simulink model "dynamic_APF"  (R2022b)
settings: Solver=VariableStepAuto  StartTime=0.0  StopTime=inf  RelTol=1e-3
InitFcn:
  | %% INITIALIZATION
  | 
  | %% UAV PARAMETERS
  | 
  | mass = 1.2;
  | Ib = diag([1.2416 1.2416 2*1.2416]);
  | 
  | %% SAMPLING TIME
  | Ts=0.001;
  | 
  | %% PLANNER
  | t_iniz = 0;
  | ttot=20; %duration
  | tdead=10; %dead time to evaluate the steady-state
  | tot_time = ttot + tdead;
  | t1=linspace(0,ttot,round(ttot/Ts));
  | t=linspace(0,ttot+tdead,round(ttot/Ts)+round(tdead/Ts));
  | p= zeros(4,length(t1)); dot_p= zeros(4,length(t1)); ddot_p= zeros(4,length(t1));
  | p_d= zeros(4,length(t)); dot_p_d= zeros(4,length(t)); ddot_p_d= zeros(4,length(t));
  | %Initial and final conditions
  | x0= 0; xf=1; dot_x0= 0; dot_xf=0; ddot_x0=0; ddot_xf=0; dddot_x0 = 0; dddot_xf = 0;
  | y0= 0; yf=1; dot_y0= 0; dot_yf=0; ddot_y0=0; ddot_yf=0; dddot_y0 = 0; dddot_yf = 0;
  | z0= -1; zf=-4; dot_z0= 0; dot_zf=0; ddot_z0=0; ddot_zf=0; dddot_z0 = 0; dddot_zf = 0;
  | psi0 = 0;
  | psif=deg2rad(20); dot_psi0= 0; dot_psif=0; ddot_psi0=0; ddot_psif=0; dddot_psi0 = 0; dddot_psif = 0;
  | p0=[x0,y0,z0,psi0]; dot_p0=[dot_x0,dot_y0,dot_z0,dot_psi0]; ddot_p0=[ddot_x0,ddot_y0,ddot_z0,ddot_psi0]; dddot_p0=[dddot_x0,dddot_y0,dddot_z0,dddot_psi0];
  | pf=[xf,yf,zf,psif]; dot_pf=[dot_xf,dot_yf,dot_zf,dot_psif]; ddot_pf=[ddot_xf,ddot_yf,ddot_zf,ddot_psif]; dddot_pf=[dddot_xf,dddot_yf,dddot_zf,dddot_psif];
  | %5-th order polynomial
  | a0=zeros(1,4); a1=zeros(1,4); a2=zeros(1,4); a3=zeros(1,4); a4=zeros(1,4); a5=zeros(1,4); a6 = zeros(1,4); a7 = zeros(1,4);
  | 
  | for j=1:4
  |     A = [t_iniz^7, t_iniz^6, t_iniz^5, t_iniz^4, t_iniz^3, t_iniz^2, t_iniz, 1;
  |         ttot^7, ttot^6, ttot^5, ttot^4, ttot^3, ttot^2, ttot, 1;
  |         7*t_iniz^6, 6*t_iniz^5, 5*t_iniz^4, 4*t_iniz^3, 3*t_iniz^2, 2*t_iniz, 1, 0;
  |         7*ttot^6, 6*ttot^5, 5*ttot^4, 4*ttot^3, 3*ttot^2, 2*ttot, 1, 0;
  |         42*t_iniz^5, 30*t_iniz^4, 20*t_iniz^3, 12*t_iniz^2, 6*t_iniz, 2, 0, 0;
  |         42*ttot^5, 30*ttot^4, 20*ttot^3, 12*ttot^2, 6*ttot, 2, 0, 0;
  |         210*t_iniz^4, 120*t_iniz^3, 60*t_iniz^2, 24*t_iniz, 6, 0, 0, 0;
  |         210*ttot^4, 120*ttot^3, 60*ttot^2, 24*ttot, 6, 0, 0, 0];
  |     b = [p0(j) pf(j) dot_p0(j) dot_pf(j) ddot_p0(j) ddot_pf(j) dddot_p0(j) dddot_pf(j)]';
  |     a_temp = A\b;
  |     a7(j) = a_temp(1);
  |     a6(j) = a_temp(2);
  |     a5(j) = a_temp(3);
  |     a4(j) = a_temp(4);
  |     a3(j) = a_temp(5);
  |     a2(j) = a_temp(6);
  |     a1(j) = a_temp(7);
  |     a0(j) = a_temp(8);
  | 
  |     %trajectories
  |     p(j,:)=a7(j)*t1.^7 + a6(j)*t1.^6 + a5(j)*t1.^5 +a4(j)*t1.^4 +a3(j)*t1.^3 +a2(j)*t1.^2 +a1(j)*t1 +a0(j);
  |     dot_p(j,:) = 7*a7(j)*t1.^6 + 6*a6(j)*t1.^5 + 5*a5(j)*t1.^4 +4*a4(j)*t1.^3 +3*a3(j)*t1.^2 +2*a2(j)*t1 +a1(j);
  |     ddot_p(j,:) = 42*a7(j)*t1.^5 + 30*a6(j)*t1.^4 + 5*4*a5(j)*t1.^3 +4*3*a4(j)*t1.^2 +3*2*a3(j)*t1 +2*a2(j);
  |     %addition of the stead-state terms
  |     p_d(j,:)=[p(j,:) zeros(1,round(tdead/Ts))+pf(j)];
  |     dot_p_d(j,:)=[dot_p(j,:) zeros(1,round(tdead/Ts))+dot_pf(j)];
  |     ddot_p_d(j,:)=[ddot_p(j,:) zeros(1,round(tdead/Ts))+ddot_pf(j)];
  | end
  | %data for Simulink
  | %pos_0 = [x0 y0 z0];
  | pos_0 = [0 0 0];
  | lin_vel_0 = [dot_x0 dot_y0 dot_z0];
  | w_bb_0 = [0 0 0];
  | csi_d=p_d(1:3,:); dot_csi_d=dot_p_d(1:3,:); ddot_csi_d=ddot_p_d(1:3,:);
  | psi_d=p_d(4,:); dot_psi_d=dot_p_d(4,:); ddot_psi_d=ddot_p_d(4,:);
undefined symbols (not defined in the file): k_att, k_rep, kp, kr, kv, kw
libraries: robotcorelib x1, simulink x1, uavutilslib x1
settings Model: Creator=fabioruggiero  LastModifiedBy=stefa
settings OptimizationCC: ReuseModelBlockBuffer=on
settings ModelReferenceCC: EnableRefExpFcnMdlSchedulingChecks=on

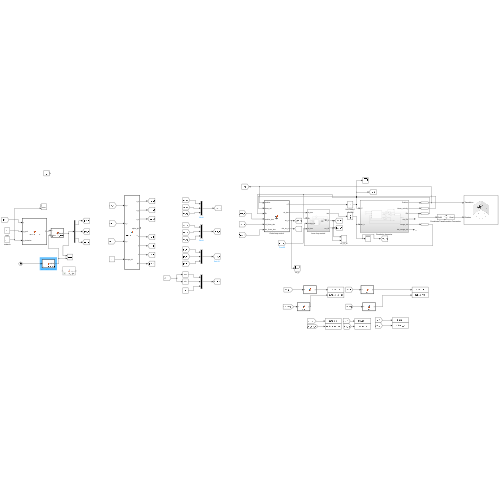
[thumbnail: Simulink's stored preview of the top-level diagram]
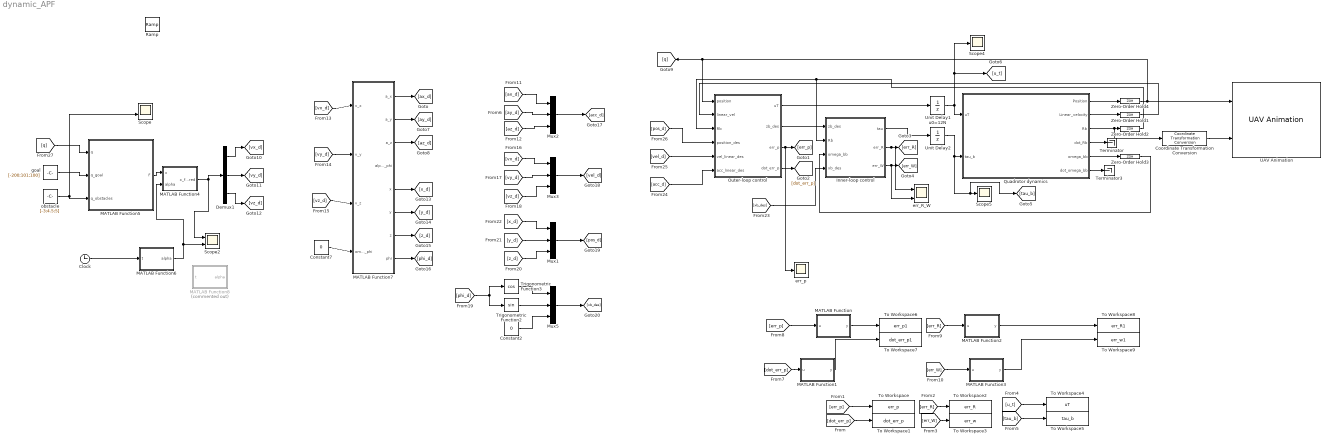
== system dynamic_APF ==
  Clock : Clock
  Constant2 : Constant  Value=0
  Constant7 : Constant  Value=0
  Coordinate Transformation Conversion : robotcorelib/Coordinate Transformation Conversion  InputRepresentation=Rotation Matrix  InputEulerSequence=ZYX  ShowTrVecInputPort=on  OutputRepresentation=Quaternion  OutputEulerSequence=ZYX  ShowTrVecOutputPort=on  SimulateUsing=Interpreted execution
  Demux1 : Demux  Outputs=3
  Inner-loop control : Subsystem
  MATLAB Function : MATLAB Function  TreatAsAtomicUnit=on
  MATLAB Function1 : MATLAB Function  TreatAsAtomicUnit=on
  MATLAB Function2 : MATLAB Function  TreatAsAtomicUnit=on
  MATLAB Function3 : MATLAB Function  TreatAsAtomicUnit=on
  MATLAB Function4 : MATLAB Function  TreatAsAtomicUnit=on
  MATLAB Function5 : MATLAB Function  TreatAsAtomicUnit=on
  MATLAB Function6 : MATLAB Function  TreatAsAtomicUnit=on
  MATLAB Function7 : MATLAB Function  TreatAsAtomicUnit=on
  MATLAB Function8 : MATLAB Function  Commented=on  TreatAsAtomicUnit=on
  Mux{1..3,5} (4 alike) : Mux  Inputs=3
  Outer-loop control : MATLAB Function  TreatAsAtomicUnit=on
  Quadrotor dynamics : Subsystem
  Ramp : simulink/Sources/Ramp  slope=1  start=0  InitialOutput=0
  Scope : Scope  NumInputPorts=2
  Scope2 : Scope  NumInputPorts=2
  Scope4 : Scope
  Scope5 : Scope
  Terminator : Terminator
  Terminator3 : Terminator
  To Workspace : ToWorkspace  VariableName=err_p  SaveFormat=Timeseries  SampleTime=-1
  To Workspace1 : ToWorkspace  VariableName=dot_err_p  SaveFormat=Timeseries  SampleTime=-1
  To Workspace2 : ToWorkspace  VariableName=err_R  SaveFormat=Timeseries  SampleTime=-1
  To Workspace3 : ToWorkspace  VariableName=err_w  SaveFormat=Timeseries  SampleTime=-1
  To Workspace4 : ToWorkspace  VariableName=uT  SaveFormat=Timeseries  SampleTime=-1
  To Workspace5 : ToWorkspace  VariableName=tau_b  SaveFormat=Timeseries  SampleTime=-1
  To Workspace6 : ToWorkspace  VariableName=err_p1  SaveFormat=Timeseries  SampleTime=-1
  To Workspace7 : ToWorkspace  VariableName=dot_err_p1  SaveFormat=Timeseries  SampleTime=-1
  To Workspace8 : ToWorkspace  VariableName=err_R1  SaveFormat=Timeseries  SampleTime=-1
  To Workspace9 : ToWorkspace  VariableName=err_w1  SaveFormat=Timeseries  SampleTime=-1
  Trigonometric Function2 : Trigonometry
  Trigonometric Function3 : Trigonometry  Operator=cos
  UAV Animation : uavutilslib/UAV Animation  UAVType=Multirotor  UAVSize=1  InertialZDirection=Down  SampleTime=0.01
  Unit Delay1 u0=12N : UnitDelay  InitialCondition=11.77  SampleTime=Ts
  Unit Delay2 : UnitDelay  InitialCondition=[0 0 0]  SampleTime=Ts
  Zero-Order Hold{1..4} (4 alike) : ZeroOrderHold  SampleTime=Ts
  err_R_W : Scope  NumInputPorts=2
  err_p : Scope
  goal : Constant  Value=[-200;101;100]
  obstacle : Constant  Value=[-3;4.5;5]
  wires:
  Outer-loop control/1(uT) -> Unit Delay1 u0=12N/1
  Unit Delay1 u0=12N/1 -> Quadrotor dynamics/1(uT), Scope4/1, [u_t]
  Quadrotor dynamics/1(Position) -> Zero-Order Hold4/1
  Quadrotor dynamics/2(Linear_velocity) -> Zero-Order Hold1/1
  Quadrotor dynamics/3(Rb) -> Coordinate Transformation Conversion/1, Zero-Order Hold2/1
  Quadrotor dynamics/5(omega_bb) -> Zero-Order Hold3/1
  Zero-Order Hold1/1 -> Outer-loop control/2(linear_vel)
  Zero-Order Hold2/1 -> Outer-loop control/3(Rb), Inner-loop control/2(Rb)
  Quadrotor dynamics/4(dot_Rb) -> Terminator/1
  Outer-loop control/3(err_p) -> err_p/1, [err_p]
  Outer-loop control/4(dot_err_p) -> [dot_err_p]
  Quadrotor dynamics/6(dot_omega_bb) -> Terminator3/1
  Coordinate Transformation Conversion/1 -> UAV Animation/2
  Outer-loop control/2(zb_des) -> Inner-loop control/1(zb_des)
  Zero-Order Hold3/1 -> Inner-loop control/3(omega_bb)
  Inner-loop control/1(tau) -> Unit Delay2/1
  [dot_err_p] -> To Workspace1/1
  [err_p] -> To Workspace/1
  Inner-loop control/2(err_R) -> err_R_W/1, [err_R]
  Inner-loop control/3(err_W) -> err_R_W/2, [err_W]
  [err_R] -> To Workspace2/1
  [err_W] -> To Workspace3/1
  Unit Delay2/1 -> [tau_b], Scope5/1, Quadrotor dynamics/2(tau_b)
  [u_t] -> To Workspace4/1
  [tau_b] -> To Workspace5/1
  [err_R] -> MATLAB Function2/1(u)
  [dot_err_p] -> MATLAB Function1/1(u)
  [err_p] -> MATLAB Function/1(u)
  [err_W] -> MATLAB Function3/1(u)
  MATLAB Function/1(y) -> To Workspace6/1
  MATLAB Function1/1(y) -> To Workspace7/1
  MATLAB Function2/1(y) -> To Workspace8/1
  MATLAB Function3/1(y) -> To Workspace9/1
  obstacle/1 -> Scope/2, MATLAB Function5/3(q_obstacles)
  Zero-Order Hold4/1 -> UAV Animation/1, [q], Outer-loop control/1(position)
  goal/1 -> MATLAB Function5/2(q_goal)
  Constant2/1 -> Mux5/3
  Trigonometric Function3/1 -> Mux5/1
  Trigonometric Function2/1 -> Mux5/2
  Constant7/1 -> MATLAB Function7/4(omega_phi)
  MATLAB Function7/1(a_x) -> [ax_d]
  MATLAB Function7/2(a_y) -> [ay_d]
  MATLAB Function7/3(a_z) -> [az_d]
  [ay_d] -> Mux2/2
  [ax_d] -> Mux2/1
  [az_d] -> Mux2/3
  Demux1/1 -> [vx_d]
  Demux1/2 -> [vy_d]
  Demux1/3 -> [vz_d]
  [vx_d] -> MATLAB Function7/1(v_x)
  [vy_d] -> MATLAB Function7/2(v_y)
  [vz_d] -> MATLAB Function7/3(v_z)
  [vx_d] -> Mux3/1
  [vy_d] -> Mux3/2
  [vz_d] -> Mux3/3
  MATLAB Function7/5(x) -> [x_d]
  MATLAB Function7/6(y) -> [y_d]
  MATLAB Function7/7(z) -> [z_d]
  MATLAB Function7/8(phi) -> [phi_d]
  [phi_d] -> Trigonometric Function2/1, Trigonometric Function3/1
  [z_d] -> Mux1/3
  [y_d] -> Mux1/2
  [x_d] -> Mux1/1
  Mux2/1 -> [acc_d]
  Mux3/1 -> [vel_d]
  Mux1/1 -> [pos_d]
  Mux5/1 -> [xb_des]
  [xb_des] -> Inner-loop control/4(xb_des)
  [acc_d] -> Outer-loop control/6(acc_linear_des)
  [vel_d] -> Outer-loop control/5(vel_linear_des)
  [pos_d] -> Outer-loop control/4(position_des)
  [q] -> MATLAB Function5/1(q)
  MATLAB Function5/1(F) -> MATLAB Function4/1(x)
  MATLAB Function4/1(x_filtered) -> Demux1/1, Scope2/1
  Clock/1 -> MATLAB Function6/1(t)
  MATLAB Function6/1(alpha) -> Scope2/2, MATLAB Function4/2(alpha)

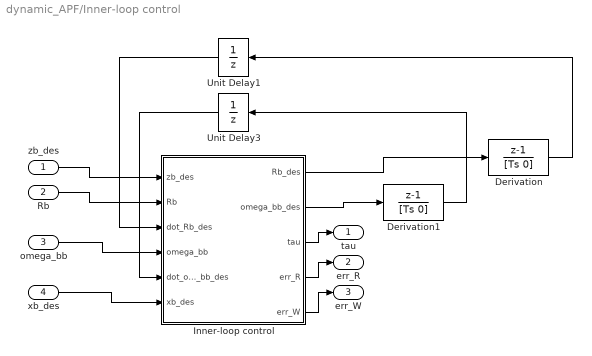
== system dynamic_APF/Inner-loop control ==
  zb_des : Inport
  Rb : Inport  Port=2
  omega_bb : Inport  Port=3
  xb_des : Inport  Port=4
  Derivation : DiscreteTransferFcn  Numerator=[1 -1]  Denominator=[Ts 0]  InitialStates=[1 0 0;0 1 0;0 0 1]  SampleTime=Ts
  Derivation1 : DiscreteTransferFcn  Numerator=[1 -1]  Denominator=[Ts 0]  InitialStates=[0 0 0]  SampleTime=Ts
  Inner-loop control : MATLAB Function  TreatAsAtomicUnit=on
  Unit Delay1 : UnitDelay  InitialCondition=eye(3)  SampleTime=Ts
  Unit Delay3 : UnitDelay  InitialCondition=[0 0 0]  SampleTime=Ts
  tau : Outport
  err_R : Outport  Port=2
  err_W : Outport  Port=3
  wires:
  xb_des/1 -> Inner-loop control/6(xb_des)
  Inner-loop control/4(err_R) -> err_R/1
  Rb/1 -> Inner-loop control/2(Rb)
  Inner-loop control/3(tau) -> tau/1
  Unit Delay1/1 -> Inner-loop control/3(dot_Rb_des)
  Derivation1/1 -> Unit Delay3/1
  Inner-loop control/5(err_W) -> err_W/1
  Unit Delay3/1 -> Inner-loop control/5(dot_omega_bb_des)
  Derivation/1 -> Unit Delay1/1
  zb_des/1 -> Inner-loop control/1(zb_des)
  omega_bb/1 -> Inner-loop control/4(omega_bb)
  Inner-loop control/1(Rb_des) -> Derivation/1
  Inner-loop control/2(omega_bb_des) -> Derivation1/1

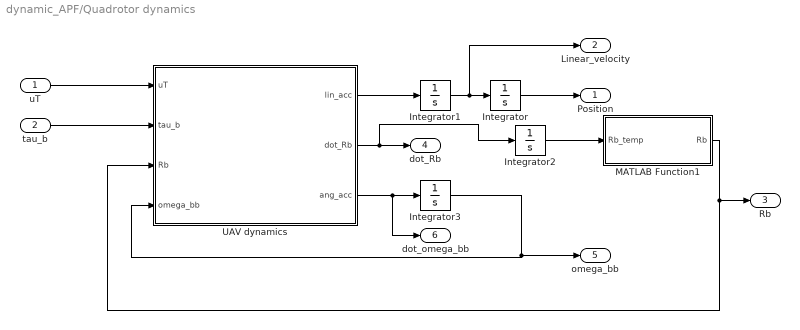
== system dynamic_APF/Quadrotor dynamics ==
  uT : Inport
  tau_b : Inport  Port=2
  Integrator : Integrator  InitialCondition=pos_0
  Integrator1 : Integrator  InitialCondition=lin_vel_0
  Integrator2 : Integrator  InitialCondition=[1 0 0; 0 1 0;0 0 1]
  Integrator3 : Integrator  InitialCondition=w_bb_0
  MATLAB Function1 : MATLAB Function  TreatAsAtomicUnit=on
  UAV dynamics : MATLAB Function  TreatAsAtomicUnit=on
  Position : Outport
  Linear_velocity : Outport  Port=2
  Rb : Outport  Port=3
  dot_Rb : Outport  Port=4
  omega_bb : Outport  Port=5
  dot_omega_bb : Outport  Port=6
  wires:
  tau_b/1 -> UAV dynamics/2(tau_b)
  Integrator/1 -> Position/1
  UAV dynamics/3(ang_acc) -> dot_omega_bb/1, Integrator3/1
  UAV dynamics/1(lin_acc) -> Integrator1/1
  uT/1 -> UAV dynamics/1(uT)
  Integrator1/1 -> Linear_velocity/1, Integrator/1
  Integrator3/1 -> UAV dynamics/4(omega_bb), omega_bb/1
  UAV dynamics/2(dot_Rb) -> Integrator2/1, dot_Rb/1
  MATLAB Function1/1(Rb) -> Rb/1, UAV dynamics/3(Rb)
  Integrator2/1 -> MATLAB Function1/1(Rb_temp)

== matlab function dynamic_APF/MATLAB Function2 ==
  data: u input; y output
function y = fcn(u)

y = norm(u);

== matlab function dynamic_APF/MATLAB Function3 ==
  data: u input; y output
function y = fcn(u)

y = norm(u);

== matlab function dynamic_APF/MATLAB Function4 ==
  settings: updateMethod=DISCRETE
  data: x input; x_filtered output; alpha input
function x_filtered = exponential_moving_average_vector(x, alpha)
    % Funzione per calcolare la media mobile esponenziale di un vettore colonna 3x1.
    % x: vettore colonna di ingresso 3x1
    % alpha: fattore di smorzamento (0 < alpha < 1)
    % x_filtered: vettore colonna filtrato 3x1
%E' lo stesso filtro che abbiamo fatto con Manfredi, la differenza è che
%alpha è tempo variante, varia in funzione esponenziale con il tempo. Se
%allontano l ostacolo nn ho problemi, tanto la Fmax dipende dai
%coefficienti, ma se vario i coefficienti posso dover ritararre il filtro(E' stato inserito per diminuire la trust iniziale)
    % Verifica che l'input x sia un vettore colonna 3x1
    if ~isequal(size(x), [3, 1])
        error('L''input x deve essere un vettore colonna 3x1.');
    end
    
    % Inizializza la variabile persistente
    persistent x_filtered_prev
    
    % Se è la prima chiamata, inizializza la variabile persistente
    if isempty(x_filtered_prev)
        x_filtered_prev = [0;0;0];
    end
    
    % Applica il filtro a media mobile esponenziale elemento per elemento
    x_filtered = (1 - alpha) * x_filtered_prev + alpha * x;
    
    % Aggiorna la variabile persistente
    x_filtered_prev = x_filtered;
end

== matlab function dynamic_APF/MATLAB Function5 ==
  data: q input; F output; q_goal input; q_obstacles input; k_att parameter; k_rep parameter
function F  = calculate_force(q, q_goal, q_obstacles, k_att, k_rep)
% Funzione per calcolare la forza totale F(q) utilizzando il metodo dei potenziali artificiali
% 
% Inputs:
%   q - Posizione attuale del UAV (3x1 vettore)
%   q_goal - Posizione del goal (3x1 vettore)
%   q_obstacles - Posizioni degli ostacoli (3xn matrice, dove n è il numero di ostacoli)
%   k_att - Coefficiente di attrazione (scalare)
%   k_rep - Coefficiente di repulsione (scalare)
%   d0 - Distanza di influenza degli ostacoli (scalare)
% 
% Output:
%   F - Forza totale (3x1 vettore)
q=-q;
k_a=k_att;

d0=2.5;
e_pos = q_goal - q;
%Ua_q= 1/2*k_att*norm(e_pos)
if(norm(e_pos)<1)
    f_a = k_a * e_pos;
else
    f_a = k_a * e_pos/norm(e_pos);
end
gamma=3;
 % Inizializza la forza repulsiva
F_rep = zeros(3, 1);

% Calcola la forza repulsiva per ciascun ostacolo
for i = 1:size(q_obstacles, 2)
    q_obs = q_obstacles(:, i);
    dist = norm(q - q_obs);
    
    if dist <= d0
        eta_q = dist;
        eta_q0 = d0;
        grad_eta_q = (q - q_obs) / dist;
        
        F_rep = F_rep + (k_rep/(eta_q^2))*(1/eta_q - 1/eta_q0)^(gamma-1) * grad_eta_q;
    end
end
F = -f_a - F_rep;
end

== matlab function dynamic_APF/MATLAB Function6 ==
  data: t input; alpha output
function alpha = calculate_alpha(t)
    % Calcola il valore di alpha in base all'istante temporale t
    
    % Define initial and final alpha values
    alpha_initial = 0.0000005;
    alpha_final = 0.5;
    
    % Define the time duration over which alpha should reach final value
    time_to_increase = 10;  % Increase alpha over 10 seconds
    alpha = alpha_initial * (100*t / 2)^2;
    % Calculate alpha based on a combination of slow start and faster growth
%     if t <= 2  % Slow start for the first 2 seconds
%         alpha = alpha_initial * (t / 2)^2;  % Quadratic ramp up
%     else
%         alpha = alpha_initial + (alpha_final - alpha_initial) * ((t - 2) / (time_to_increase - 2));
%     end
    
    % Ensure alpha is within bounds
    alpha = max(min(alpha, alpha_final), alpha_initial);
end

== matlab function dynamic_APF/MATLAB Function7 ==
  settings: updateMethod=DISCRETE
  data: a_x output; a_y output; a_z output; alpha_phi output; x output; v_x input; y output; v_y input; v_z input; omega_phi input; z output; phi output; Ts parameter double
function [a_x, a_y, a_z, alpha_phi, x, y, z, phi] = calculate_state(v_x, v_y, v_z, omega_phi, Ts)
    % Calcola le posizioni e le accelerazioni a partire dalle velocità
    % Inizializza le variabili persistenti
    persistent x_prev y_prev z_prev phi_prev
    persistent v_x_prev v_y_prev v_z_prev omega_phi_prev
    dt=Ts;
    % Se è la prima chiamata, inizializza le variabili persistenti
    if isempty(x_prev)
        x_prev = 0;
        y_prev = 0;
        z_prev = 0;
        phi_prev = 0;
        v_x_prev = 0;
        v_y_prev = 0;
        v_z_prev = 0;
        omega_phi_prev = 0;
    end
    
    % Calcola le posizioni integrando le velocità
    x = x_prev + v_x * dt;
    y = y_prev + v_y * dt;
    z = z_prev + v_z * dt;
    phi = phi_prev + omega_phi * dt;
    
    % Calcola le accelerazioni derivando le velocità
    a_x = (v_x - v_x_prev) / dt;
    a_y = (v_y - v_y_prev) / dt;
    a_z = (v_z - v_z_prev) / dt;
    alpha_phi = (omega_phi - omega_phi_prev) / dt;
    
    % Aggiorna le variabili persistenti
    x_prev = x;
    y_prev = y;
    z_prev = z;
    phi_prev = phi;
    v_x_prev = v_x;
    v_y_prev = v_y;
    v_z_prev = v_z;
    omega_phi_prev = omega_phi;
end

== matlab function dynamic_APF/MATLAB Function8 ==
  data: t input; alpha output
function alpha = calculate_alpha(t)
    % Calcola il valore di alpha in base all'istante temporale t
    
    % Define initial and final alpha values
    alpha_initial = 0.05;
    alpha_final = 1;
    
    % Define the time duration over which alpha should increase
    time_to_increase = 5;  % Increase alpha over 10 seconds
    
    % Calculate alpha based on linear interpolation
    if t <= time_to_increase
        alpha = alpha_initial + (alpha_final - alpha_initial) * (t / time_to_increase);
    else
        alpha = alpha_final;
    end
end

== matlab function dynamic_APF/MATLAB Function ==
  data: u input; y output
function y = fcn(u)

y = norm(u);

== matlab function dynamic_APF/Quadrotor dynamics/UAV dynamics ==
  data: uT input size=1; tau_b input size=3; lin_acc output size=3; Rb input size=[3,3]; omega_bb input size=3; dot_Rb output size=[3,3]; ang_acc output size=3; mass parameter size=1; Ib parameter size=[3,3]
function [lin_acc, dot_Rb, ang_acc] = fcn(uT,tau_b,Rb,omega_bb,mass, Ib)

lin_acc = 9.81*[0 0 1]'-(uT/mass)*Rb*[0 0 1]';
dot_Rb = Rb*skew(omega_bb);
ang_acc = inv(Ib)*(-skew(omega_bb)*Ib*omega_bb + tau_b);

end

function S = skew(v)
if(numel(v)~= 1)
S= [0 -v(3) v(2); 
    v(3) 0 -v(1);
    -v(2) v(1) 0];
else
S= zeros(3);
end
end

== matlab function dynamic_APF/Outer-loop control ==
  data: position input size=3; uT output size=1; linear_vel input size=3; Rb input size=[3,3]; zb_des output size=3; mass parameter size=1; position_des input size=3; vel_linear_des input size=3; acc_linear_des input size=3; err_p output size=3; dot_err_p output size=3; kp parameter; kv parameter
function [uT, zb_des, err_p, dot_err_p] = fcn(position, linear_vel, Rb, mass, ...
    position_des, vel_linear_des, acc_linear_des, kp, kv)

%% WRITE HERE THE OUTER-LOOP CONTROL
% position: linear position measure
% linear_vel: linear velocity measure
% Rb: current rotation matrix
% mass: mass of the UAV
% positon_des: desired linear position from the planner
% vel_linear_des: desired linear velocity from the planner
% acc_linear_des: desired linear acceleration from the planner
% ---
% uT: commanded total thrust
% zb_des: desired z-axis of the body frame
% err_p: position error
% dot_err_p: time derivative of the positon error

%% OUTER-LOOP CONTROL
g = 9.81;
err_p = position - position_des;
dot_err_p = linear_vel - vel_linear_des;


%NON SO COME CHIAMARLA se avete fantasia diamogli un nome decente
num = -kp * err_p - kv * dot_err_p - mass * g * [0; 0; 1] + mass * acc_linear_des;

uT = ((-num')* Rb * [0; 0; 1]);  

zb_des = - num / norm(num);

== matlab function dynamic_APF/Inner-loop control/Inner-loop control ==
  data: Rb_des output size=[3,3]; omega_bb_des output size=3; tau output size=3; zb_des input size=3; Rb input size=[3,3]; dot_Rb_des input size=[3,3]; omega_bb input size=3; dot_omega_bb_des input size=3; xb_des input size=3; Ib parameter size=[3,3]; err_R output size=3; err_W output size=3; kw parameter; kr parameter
function [Rb_des,omega_bb_des,tau,err_R,err_W] = fcn(zb_des,Rb,dot_Rb_des,omega_bb,dot_omega_bb_des,xb_des,Ib, kw, kr)

%% WRITE HERE THE INNER-LOOP CONTROL
% zb_des: desired z-axis of the body frame
% Rb: current rotation matrix
% dot_Rb_des: time-derivative of the desired rotation matrix
% omega_bb: current angular velocity expressed in the body frame
% dot_omega_bb_des: desired angular acceleration expressed in the body
% frame
% xb_des: desired x-axis of the body frame form the planner
% Ib: inertia matrix of the UAV with respect to the body frame
% ---
% Rb_des: desired rotation matrix
% omega_bb_des: desired angular velocity expressed in the body frame (given
% below as a hint)
% tau: commanded control torque
% err_R: rotational error in SO(3)
% err_W: angular velocity error in SO(3)

yb_des=( skew(zb_des) * xb_des) / norm( ( skew(zb_des) * xb_des) );

Rb_des=[skew(yb_des)*zb_des yb_des zb_des];

err_R= 1/2 * wedge( (Rb_des') * Rb - (Rb') * Rb_des);

omega_bb_des = wedge(Rb_des'*dot_Rb_des);

err_W=omega_bb - (Rb') * Rb_des * omega_bb_des; 

tau=-kr * err_R - kw * err_W + skew(omega_bb) * Ib * omega_bb - Ib * (skew(omega_bb) * (Rb') * Rb_des * omega_bb_des - (Rb') * Rb_des * dot_omega_bb_des);
end

function S = skew(v)
if(numel(v)~= 1)
S= [0 -v(3) v(2); 
    v(3) 0 -v(1);
    -v(2) v(1) 0];
else
S= zeros(3);
end
end

function v = wedge(S)
v1 = S(3,2);
v2 = S(1,3);
v3 = S(2,1);
v = [v1 v2 v3]';
end

== matlab function dynamic_APF/Quadrotor dynamics/MATLAB Function1 ==
  data: Rb_temp input; Rb output
function Rb = fcn(Rb_temp)
    [U,S,V] = svd(Rb_temp);
    sigma = det(U*V');
    S_ = diag([1 1 sigma]);

    Rb = U*S_*V';
end

== matlab function dynamic_APF/MATLAB Function1 ==
  data: u input; y output
function y = fcn(u)

y = norm(u);
